simulink model "prattico_simscape_phase_b"  (R2025b)
settings: Solver=ode23t  StartTime=0.0  StopTime=1  MaxStep=3e-6  RelTol=1e-4  AbsTol=1e-5
libraries: fl_lib x24, nesl_utility x14, simulink x8, batteryecm_lib x1, slpidlib x1, ee_lib x1
settings Model: Creator=oakir  LastModifiedBy=oakir
settings DataIOCC: SignalLogging=off  ReturnWorkspaceOutputs=off

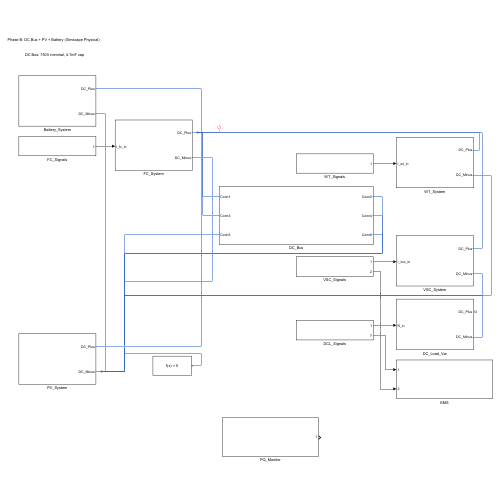
[thumbnail: Simulink's stored preview of the top-level diagram]
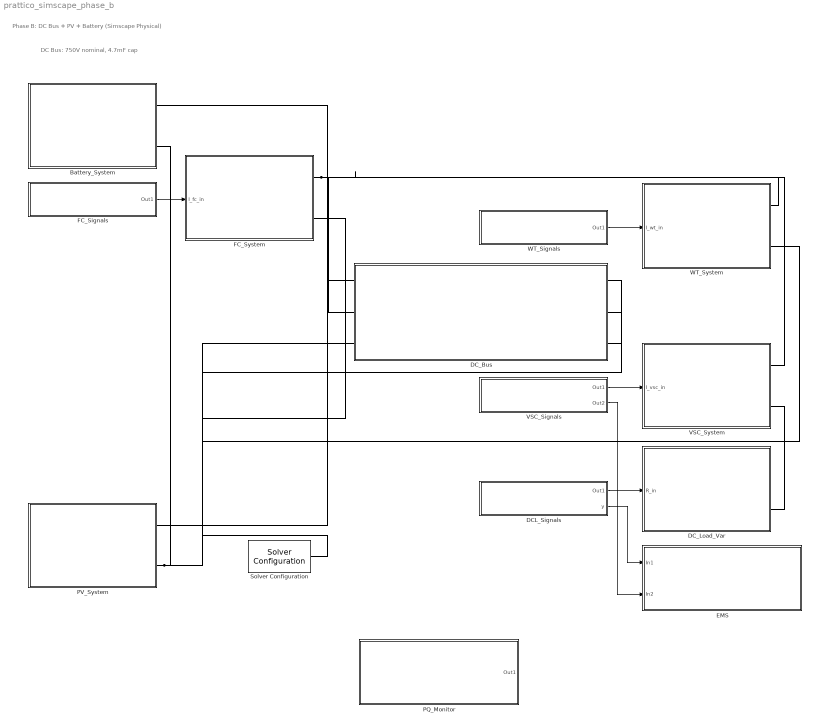
== system prattico_simscape_phase_b ==
  note: DC Bus: 750V nominal, 4.7mF cap
  note: Phase B: DC Bus + PV + Battery (Simscape Physical)
  Battery_System : Subsystem
  DCL_Signals : Subsystem
  DC_Bus : Subsystem
  DC_Load_Var : Subsystem
  EMS : Subsystem
  FC_Signals : Subsystem
  FC_System : Subsystem
  PQ_Monitor : Subsystem
  PV_System : Subsystem
  Solver Configuration : nesl_utility/Solver Configuration  PhysicalDomain=network_engine_domain  SubClassName=solver  LeftPortType=input  RightPortType=generic  Tones=[]  Harmonics=[]  SimulateNoise=off  Profile=off  UseLocalSampling=off  EnableSwitchedLinearOptims=on  FrequencyDomain=off  UseCCode=off  RelTol=0.001  AbsTol=0.001  MinStep=1e-09  ToWorkspace=off  RevertToSquareIcSolve=off  NumHomotopyIterations=100  PhasorMode=off  PhasorModeNumHarmonics=1  ConsistencySolver=NEWTON_XTOL_AFTER_FTOL  IndexReductionMethod=DerivativeReplacement  DoDC=off  ResidualTolerance=1e-09  ConsistencyTolSource=GLOBAL  ConsistencyAbsTol=0.001  ConsistencyRelTol=0.001  ConsistencyTolFactor=0.001  UseLocalSolver=off  LocalSolverChoice=NE_BACKWARD_EULER_ADVANCER  ResolveIndetEquations=on  FunctionEvalNumThread=1  LocalSolverSampleTime=0.001  DoFixedCost=off  MaxNonlinIter=3  MaxModeIter=2  ComputeImpulses=off  ImpulseIterations=2  LinearAlgebra=auto  LinearAlgebraNumThread=0  EquationFormulation=NE_TIME_EF  DelaysMemoryBudget=1024  AutomaticFiltering=on  FilteringTimeConstant=0.001  PartitionStorageMethod=AS_NEEDED  PartitionMemoryBudget=1024  PartitionMethod=ROBUST  MultibodyUseLocalSolver=off  MultibodyLocalSolverChoice=ODE1  MultibodyLocalSolverSampleTime=0.001
  VSC_Signals : Subsystem
  VSC_System : Subsystem
  WT_Signals : Subsystem
  WT_System : Subsystem
  wires:
  FC_Signals/1(Out1) -> FC_System/1(I_fc_in)
  DCL_Signals/2(y) -> EMS/1(In1)
  DCL_Signals/1(Out1) -> DC_Load_Var/1(R_in)
  WT_Signals/1(Out1) -> WT_System/1(I_wt_in)
  VSC_Signals/2(Out2) -> EMS/2(In2)
  VSC_Signals/1(Out1) -> VSC_System/1(I_vsc_in)
  connections:
  FC_System/RConn1 -- VSC_System/RConn1 -- Battery_System/RConn1 -- WT_System/RConn1 -- DC_Bus/LConn2 -- DC_Bus/LConn1 -- PV_System/RConn1
  DC_Bus/RConn2 -- Solver Configuration/RConn1 -- PV_System/RConn2 -- FC_System/RConn2 -- WT_System/RConn2 -- VSC_System/RConn2 -- DC_Load_Var/RConn2 -- Battery_System/RConn2 -- DC_Bus/RConn3 -- DC_Bus/LConn3 -- DC_Bus/RConn1

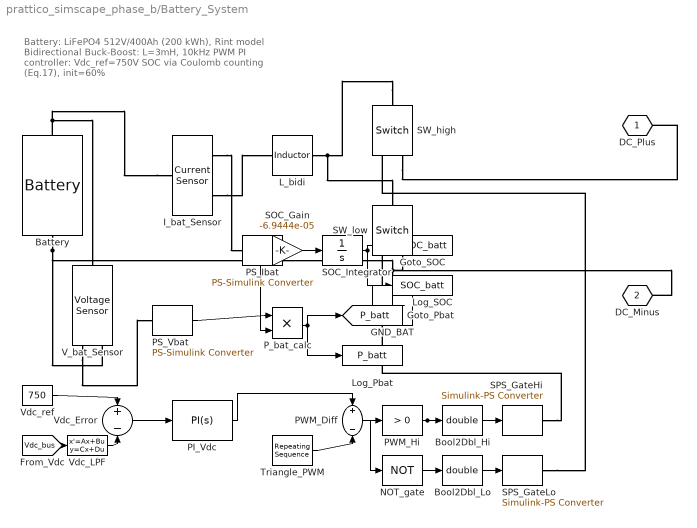
== system prattico_simscape_phase_b/Battery_System ==
  note: Battery: LiFePO4 512V/400Ah (200 kWh), Rint model
      | Bidirectional Buck-Boost: L=3mH, 10kHz PWM
      | PI controller: Vdc_ref=750V
      | SOC via Coulomb counting (Eq.17), init=60%
  Battery : batteryecm_lib/Battery  Vnom=512 V  prm_dir=simscape.enum.battery.prm_dir.disabled  R1_dis=2 Ohm  R1_ch=2 Ohm  R1=0.04 Ohm  prm_AH=simscape.enum.battery.prm_AH.infinite  AH=400 A*hr  V1=480 V  AH1=360 A*hr  prm_R2=simscape.enum.battery.prm_R2.disabled  R2=2000 Ohm  Tmeas=298.15 K  charge_measurement_port=simscape.enum.battery.enable.no  prm_dyn=simscape.enum.battery.prm_dyn.off  Rp1=0.005 Ohm  tau1=30 s  Rp2=0.005 Ohm  tau2=30 s  Rp3=0.005 Ohm  tau3=30 s  Rp4=0.005 Ohm  tau4=30 s  Rp5=0.005 Ohm  tau5=30 s  prm_fade=simscape.enum.battery.prm_fade.disabled  N_fade=100  AH_fade=45 A*hr  R1_fade=2.02 Ohm  R1_ch_fade=2.02 Ohm  V1_fade=10.35 V  prm_age=simscape.enum.battery.prm_age.disabled  prm_age_OCV=simscape.enum.battery.prm_age_OCV.OCV  OCV_age=0.9  SOC_age=60  Tmeas_age=298.15 K  delta_time_age_vec=[0] d  temperature_age_vec=[273] K  OCV_scaling_age=2.2134e6  OCV_offset_age=1.632e6  temp_exp_age=0.515833569 V  t_exp_age=0.75  Vnom_T2=12 V  R1_T2=2.2 Ohm  R1_T2_dis=2.2 Ohm  R1_T2_ch=2.2 Ohm  V1_T2=11.4 V  R2_T2=2200 Ohm  Rp1_T2=0.005 Ohm  tau1_T2=30 s  Rp2_T2=0.005 Ohm  tau2_T2=30 s  Rp3_T2=0.005 Ohm  tau3_T2=30 s  Rp4_T2=0.005 Ohm  tau4_T2=30 s  Rp5_T2=0.005 Ohm  tau5_T2=30 s  Tmeas2=273.15 K  thermal_port=simscape.enum.thermaleffects.omit  thermal_mass=30000 J/K  i_specify=off  i_priority=None  i=0 A  i_nominal_specify=off  i_nominal_value=1  i_nominal_unit=A  v_specify=off  v_priority=None  v=0 V  v_nominal_specify=off  v_nominal_value=1  v_nominal_unit=V  charge_specify=off  charge_priority=High  charge=50 A*hr  charge_nominal_specify=off  charge_nominal_value=1  charge_nominal_unit=A*hr  num_cycles_specify=off  num_cycles_priority=High  num_cycles=0  num_cycles_nominal_specify=off  num_cycles_nominal_value=1  num_cycles_nominal_unit=1  temperature_specify=off  temperature_priority=High  temperature=298.15 K  temperature_nominal_specify=off  temperature_nominal_value=1  temperature_nominal_unit=K
  Bool2Dbl_Hi : DataTypeConversion  OutDataTypeStr=double  SaturateOnIntegerOverflow=off  RndMeth=Floor
  Bool2Dbl_Lo : DataTypeConversion  OutDataTypeStr=double  SaturateOnIntegerOverflow=off  RndMeth=Floor
  GND_BAT : fl_lib/Electrical/Electrical Elements/Electrical Reference
  I_bat_Sensor : fl_lib/Electrical/Electrical Sensors/Current Sensor
  L_bidi : fl_lib/Electrical/Electrical Elements/Inductor  l=3e-3 H  r=0 Ohm  g=1e-9 1/Ohm  i_specify=off  i_priority=None  i=0 A  i_nominal_specify=off  i_nominal_value=1  i_nominal_unit=A  v_specify=off  v_priority=None  v=0 V  v_nominal_specify=off  v_nominal_value=1  v_nominal_unit=V  i_L_specify=off  i_L_priority=High  i_L=0 A  i_L_nominal_specify=off  i_L_nominal_value=1  i_L_nominal_unit=A
  Log_Pbat : ToWorkspace  VariableName=P_batt  SaveFormat=Timeseries  SampleTime=-1
  Log_SOC : ToWorkspace  VariableName=SOC_batt  SaveFormat=Timeseries  SampleTime=-1
  NOT_gate : Logic  Operator=NOT  AllPortsSameDT=off  OutDataTypeStr=boolean
  PI_Vdc : slpidlib/PID Controller  Controller=PI  Form=Parallel  TimeDomain=Continuous-time  UseExternalTs=off  SampleTime=-1  IntegratorMethod=Forward Euler  FilterMethod=Forward Euler  ControllerParametersSource=internal  P=0.0001  I=0.02  UseKiTs=off  D=0  UseExternalDerivativeSource=off  N=100  UseFilter=on  TunerSelectOption=Transfer Function Based (PID Tuner App)  InitialConditionSource=internal  InitialConditionForIntegrator=0.32  InitialConditionForFilter=0  DifferentiatorICPrevScaledInput=0  ExternalReset=none  TrackingMode=off  Kt=1  LimitOutput=off  SatLimitsSource=internal  UpperSaturationLimit=0.45  LowerSaturationLimit=0.05  LinearizeAsGain=on  AntiWindupMode=none  Kb=1  LimitIntegrator=off  UpperIntegratorSaturationLimit=inf  LowerIntegratorSaturationLimit=-inf  POutMin=[]  POutMax=[]  IOutMin=[]  IOutMax=[]  DOutMin=[]  DOutMax=[]  NOutMin=[]  NOutMax=[]  SumOutMin=[]  SumOutMax=[]  SaturationOutMin=[]  SaturationOutMax=[]  PParamMin=[]  PParamMax=[]  IParamMin=[]  IParamMax=[]  DParamMin=[]  DParamMax=[]  NParamMin=[]  NParamMax=[]  KbParamMin=[]  KbParamMax=[]  KtParamMin=[]  KtParamMax=[]  KbOutMin=[]  KbOutMax=[]  KtOutMin=[]  KtOutMax=[]  IntegratorOutMin=[]  IntegratorOutMax=[]  FilterOutMin=[]  FilterOutMax=[]  SumI1OutMin=[]  SumI1OutMax=[]  SumI2OutMin=[]  SumI2OutMax=[]  SumI3OutMin=[]  SumI3OutMax=[]  SumI4OutMin=[]  SumI4OutMax=[]  SumDOutMin=[]  SumDOutMax=[]  DifferentiatorOutMin=[]  DifferentiatorOutMax=[]  FilterDiffOutCoefMin=[]  FilterDiffOutCoefMax=[]  ReciprocalOutMin=[]  ReciprocalOutMax=[]  SumDenOutMin=[]  SumDenOutMax=[]  SumNumOutMin=[]  SumNumOutMax=[]  DivideOutMin=[]  DivideOutMax=[]  UdiffTsProdOutMin=[]  UdiffTsProdOutMax=[]  NTsProdOutMin=[]  NTsProdOutMax=[]  UintegralTsProdOutMin=[]  UintegralTsProdOutMax=[]  UngainTsProdOutMin=[]  UngainTsProdOutMax=[]  ClampingZeroOutDataTypeStr=Inherit: Inherit via back propagation  ClampingZeroOutMin=[]  ClampingZeroOutMax=[]  FilterDenConstantOutDataTypeStr=Inherit: Inherit via back propagation  FilterDenConstantOutMin=[]  FilterDenConstantOutMax=[]  PCopyOutDataTypeStr=Inherit: Inherit via back propagation  PCopyOutMin=[]  PCopyOutMax=[]  NCopyOutDataTypeStr=Inherit: Inherit via back propagation  NCopyOutMin=[]  NCopyOutMax=[]  IntegratorContinuousStateAttributes=''  IntegratorStateMustResolveToSignalObject=off  IntegratorRTWStateStorageClass=Auto  FilterContinuousStateAttributes=''  FilterStateMustResolveToSignalObject=off  FilterRTWStateStorageClass=Auto  ParallelPVariant=InternalParameters  IdealPVariant=Disabled  IVariant=InternalParameters  DVariant=Disabled  IntegratorVariant=Continuous  SatVariant=Disabled  AWVariant=Passthrough  PCopyVariant=Disabled  TRVariant=Disabled  FdbkBlocksVariant=Forward  IdealPFdbkVariant=Disabled  SatFdbkVariant=Disabled  DerivativeFilterVariant=Disabled  NVariant=Disabled  NCopyVariant=Disabled_SignalSpec  FilterICVariant=Disabled  IntegratorICVariant=InternalICs  ExternalResetVariant=Disabled  TRSumVariant=Passthrough  SumFdbkVariant=Disabled  SumVariant=Sum_PI  TsampFilterVariant=InternalTs  TsampNgainVariant=Passthrough  TsampIntegralVariant=Disabled_SignalSpec  ExternalSaturationOutDataTypeStr=Inherit: Same as second input  DerivativeSourceVariant=Disabled  PreIntVariant=InternalPreInt
  PS_Ibat : nesl_utility/PS-Simulink Converter  PhysicalDomain=network_engine_domain  SubClassName=ps_output  LeftPortType=input  RightPortType=output  PseudoPeriodic=off  Frequencies=[]  VectorFormat=inherit  Unit=inherit  AffineConversion=off
  PS_Vbat : nesl_utility/PS-Simulink Converter  PhysicalDomain=network_engine_domain  SubClassName=ps_output  LeftPortType=input  RightPortType=output  PseudoPeriodic=off  Frequencies=[]  VectorFormat=inherit  Unit=inherit  AffineConversion=off
  PWM_Diff : Sum  Inputs=+-
  PWM_Hi : simulink/Logic and Bit Operations/Compare To Zero  relop=>  OutDataTypeStr=boolean
  P_bat_calc : Product
  SOC_Gain : Gain  Gain=-6.9444e-05
  SOC_Integrator : Integrator  InitialCondition=60  UpperSaturationLimit=100  LowerSaturationLimit=0
  SPS_GateHi : nesl_utility/Simulink-PS Converter  PhysicalDomain=network_engine_domain  SubClassName=ps_input  LeftPortType=input  RightPortType=output  PseudoPeriodic=off  Frequencies=[]  NoiseDistribution=none  NoiseParameters=[]  Unit=1  AffineConversion=off  FilteringAndDerivatives=provide  SimscapeFilterOrder=1  InputFilterTimeConstant=1e-7  UdotUserProvided=0
  SPS_GateLo : nesl_utility/Simulink-PS Converter  PhysicalDomain=network_engine_domain  SubClassName=ps_input  LeftPortType=input  RightPortType=output  PseudoPeriodic=off  Frequencies=[]  NoiseDistribution=none  NoiseParameters=[]  Unit=1  AffineConversion=off  FilteringAndDerivatives=provide  SimscapeFilterOrder=1  InputFilterTimeConstant=1e-7  UdotUserProvided=0
  SW_high : fl_lib/Electrical/Electrical Elements/Switch  R_closed=0.01 Ohm  G_open=1e-8 1/Ohm  Threshold=0.5  i_specify=off  i_priority=None  i=0 A  i_nominal_specify=off  i_nominal_value=1  i_nominal_unit=A  v_specify=off  v_priority=None  v=0 V  v_nominal_specify=off  v_nominal_value=1  v_nominal_unit=V
  SW_low : fl_lib/Electrical/Electrical Elements/Switch  R_closed=0.01 Ohm  G_open=1e-8 1/Ohm  Threshold=0.5  i_specify=off  i_priority=None  i=0 A  i_nominal_specify=off  i_nominal_value=1  i_nominal_unit=A  v_specify=off  v_priority=None  v=0 V  v_nominal_specify=off  v_nominal_value=1  v_nominal_unit=V
  Triangle_PWM : simulink/Sources/Repeating Sequence  rep_seq_t=[0 5e-5 1e-4]  rep_seq_y=[0 1 0]
  V_bat_Sensor : fl_lib/Electrical/Electrical Sensors/Voltage Sensor
  Vdc_Error : Sum  Inputs=+-
  Vdc_LPF : StateSpace  A=-200  B=200  D=0  InitialCondition=750
  Vdc_ref : Constant  Value=750
  DC_Plus : PMIOPort  Side=Right
  DC_Minus : PMIOPort  Port=2  Side=Right
  tag scope: P_batt=global, SOC_batt=global
  wires:
  PS_Ibat/1 -> SOC_Gain/1, P_bat_calc/2
  SOC_Gain/1 -> SOC_Integrator/1
  SOC_Integrator/1 -> [SOC_batt], Log_SOC/1
  PS_Vbat/1 -> P_bat_calc/1
  P_bat_calc/1 -> [P_batt], Log_Pbat/1
  Vdc_ref/1 -> Vdc_Error/1
  [Vdc_bus] -> Vdc_LPF/1
  Vdc_LPF/1 -> Vdc_Error/2
  Vdc_Error/1 -> PI_Vdc/1
  PI_Vdc/1 -> PWM_Diff/1
  Triangle_PWM/1 -> PWM_Diff/2
  PWM_Diff/1 -> PWM_Hi/1
  PWM_Hi/1 -> Bool2Dbl_Hi/1, NOT_gate/1
  Bool2Dbl_Hi/1 -> SPS_GateHi/1
  NOT_gate/1 -> Bool2Dbl_Lo/1
  Bool2Dbl_Lo/1 -> SPS_GateLo/1
  connections:
  I_bat_Sensor/LConn1 -- Battery/LConn1 -- V_bat_Sensor/LConn1
  I_bat_Sensor/RConn2 -- L_bidi/LConn1
  Battery/RConn1 -- V_bat_Sensor/RConn2 -- SW_low/RConn2 -- GND_BAT/LConn1 -- DC_Minus/RConn1
  SW_high/LConn1 -- L_bidi/RConn1 -- SW_low/LConn1
  SW_high/RConn2 -- DC_Plus/RConn1
  SPS_GateHi/RConn1 -- SW_low/RConn1
  SPS_GateLo/RConn1 -- SW_high/RConn1
  I_bat_Sensor/RConn1 -- PS_Ibat/LConn1
  V_bat_Sensor/RConn1 -- PS_Vbat/LConn1

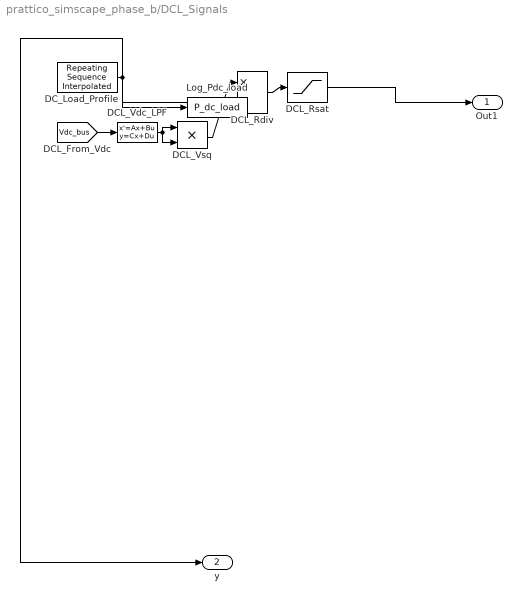
== system prattico_simscape_phase_b/DCL_Signals ==
  DCL_Rdiv : Product  Inputs=*/
  DCL_Rsat : Saturate  UpperLimit=1e6  LowerLimit=1
  DCL_Vdc_LPF : StateSpace  A=-200  B=200  D=0  InitialCondition=750
  DCL_Vsq : Product  Inputs=**
  DC_Load_Profile : simulink/Sources/Repeating Sequence Interpolated  OutValues=[1500 1500 6000 12000 12000 12000 15000 12000 10000 6000 3000 1500 1500]  TimeValues=[0 7 7.5 8.5 9 11 14 15 17 19 20 22 24]  LookUpMeth=Interpolation-Use End Values  tsamp=0.01  OutMin=[]  OutMax=[]  OutDataTypeStr=double  OutputDataTypeScalingMode=double  OutDataType=fixdt(0,8)  OutScaling=2^-10
  Log_Pdc_load : ToWorkspace  VariableName=P_dc_load  SaveFormat=Timeseries  SampleTime=-1
  Out1 : Outport
  y : Outport  Port=2
  wires:
  DC_Load_Profile/1 -> y/1, Log_Pdc_load/1, DCL_Rdiv/2
  DCL_Vsq/1 -> DCL_Rdiv/1
  DCL_Vdc_LPF/1 -> DCL_Vsq/1, DCL_Vsq/2
  [Vdc_bus] -> DCL_Vdc_LPF/1
  DCL_Rdiv/1 -> DCL_Rsat/1
  DCL_Rsat/1 -> Out1/1

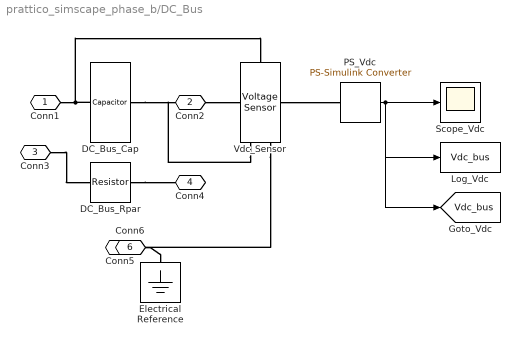
== system prattico_simscape_phase_b/DC_Bus ==
  DC_Bus_Cap : fl_lib/Electrical/Electrical Elements/Capacitor  c=4.7e-3 F  r=1e-6 Ohm  g=0 1/Ohm  i_specify=off  i_priority=None  i=0 A  i_nominal_specify=off  i_nominal_value=1  i_nominal_unit=A  v_specify=off  v_priority=None  v=750 V  v_nominal_specify=off  v_nominal_value=1  v_nominal_unit=V  vc_specify=off  vc_priority=High  vc=0 V  vc_nominal_specify=off  vc_nominal_value=1  vc_nominal_unit=V
  DC_Bus_Rpar : fl_lib/Electrical/Electrical Elements/Resistor  R=1e4 Ohm  i_specify=off  i_priority=None  i=0 A  i_nominal_specify=off  i_nominal_value=1  i_nominal_unit=A  v_specify=off  v_priority=None  v=0 V  v_nominal_specify=off  v_nominal_value=1  v_nominal_unit=V
  Electrical Reference : fl_lib/Electrical/Electrical Elements/Electrical Reference
  Log_Vdc : ToWorkspace  VariableName=Vdc_bus  SaveFormat=Timeseries  SampleTime=-1
  PS_Vdc : nesl_utility/PS-Simulink Converter  PhysicalDomain=network_engine_domain  SubClassName=ps_output  LeftPortType=input  RightPortType=output  PseudoPeriodic=off  Frequencies=[]  VectorFormat=inherit  Unit=inherit  AffineConversion=off
  Scope_Vdc : Scope
  Vdc_Sensor : fl_lib/Electrical/Electrical Sensors/Voltage Sensor
  Conn1 : PMIOPort  Side=Left
  Conn2 : PMIOPort  Port=2  Side=Right
  Conn3 : PMIOPort  Port=3  Side=Left
  Conn4 : PMIOPort  Port=4  Side=Right
  Conn5 : PMIOPort  Port=5  Side=Left
  Conn6 : PMIOPort  Port=6  Side=Right
  tag scope: Vdc_bus=global
  wires:
  PS_Vdc/1 -> Scope_Vdc/1, Log_Vdc/1, [Vdc_bus]
  connections:
  Conn3/RConn1 -- DC_Bus_Rpar/LConn1
  DC_Bus_Rpar/RConn1 -- Conn4/RConn1
  Vdc_Sensor/RConn1 -- PS_Vdc/LConn1
  Vdc_Sensor/RConn2 -- Conn6/RConn1
  DC_Bus_Cap/RConn1 -- Conn2/RConn1
  Conn1/RConn1 -- Vdc_Sensor/LConn1 -- DC_Bus_Cap/LConn1
  Conn5/RConn1 -- Electrical Reference/LConn1

== system prattico_simscape_phase_b/DC_Load_Var ==
  R_in : Inport
  SPS_R : nesl_utility/Simulink-PS Converter  PhysicalDomain=network_engine_domain  SubClassName=ps_input  LeftPortType=input  RightPortType=output  PseudoPeriodic=off  Frequencies=[]  NoiseDistribution=none  NoiseParameters=[]  Unit=1  AffineConversion=off  FilteringAndDerivatives=provide  SimscapeFilterOrder=1  InputFilterTimeConstant=0.001  UdotUserProvided=0
  VR_DC : fl_lib/Electrical/Electrical Elements/Variable Resistor  Rmin=0 Ohm  thermalEnable=false  thermal_mass=1 J/K  i_specify=off  i_priority=None  i=0 A  i_nominal_specify=off  i_nominal_value=1  i_nominal_unit=A  v_specify=off  v_priority=None  v=0 V  v_nominal_specify=off  v_nominal_value=1  v_nominal_unit=V  T_specify=off  T_priority=None  T=300 K  T_nominal_specify=off  T_nominal_value=1  T_nominal_unit=K
  DC_Plus : PMIOPort  Side=Right
  DC_Minus : PMIOPort  Port=2  Side=Right
  wires:
  R_in/1 -> SPS_R/1
  connections:
  VR_DC/LConn1 -- DC_Plus/RConn1
  VR_DC/RConn1 -- DC_Minus/RConn1

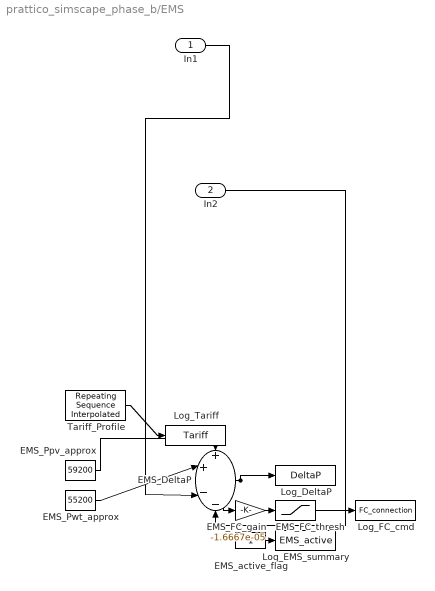
== system prattico_simscape_phase_b/EMS ==
  In1 : Inport
  In2 : Inport  Port=2
  EMS_DeltaP : Sum  Inputs=++--
  EMS_FC_gain : Gain  Gain=-1.6667e-05
  EMS_FC_thresh : Saturate  UpperLimit=1  LowerLimit=0
  EMS_Ppv_approx : Constant  Value=59200
  EMS_Pwt_approx : Constant  Value=55200
  EMS_active_flag : Constant
  Log_DeltaP : ToWorkspace  VariableName=DeltaP  SaveFormat=Timeseries  SampleTime=-1
  Log_EMS_summary : ToWorkspace  VariableName=EMS_active  SaveFormat=Timeseries  SampleTime=-1
  Log_FC_cmd : ToWorkspace  VariableName=FC_connection  SaveFormat=Timeseries  SampleTime=-1
  Log_Tariff : ToWorkspace  VariableName=Tariff  SaveFormat=Timeseries  SampleTime=-1
  Tariff_Profile : simulink/Sources/Repeating Sequence Interpolated  OutValues=[0.05 0.05 0.08 0.1 0.12 0.1 0.15 0.15 0.1 0.05]  TimeValues=[0 6 7 9 11 17 19 21 22 24]  LookUpMeth=Interpolation-Use End Values  tsamp=0.01  OutMin=[]  OutMax=[]  OutDataTypeStr=double  OutputDataTypeScalingMode=double  OutDataType=fixdt(0,8)  OutScaling=2^-10
  wires:
  EMS_Ppv_approx/1 -> EMS_DeltaP/1
  EMS_DeltaP/1 -> Log_DeltaP/1, EMS_FC_gain/1
  Tariff_Profile/1 -> Log_Tariff/1
  In2/1 -> EMS_DeltaP/4
  EMS_FC_gain/1 -> EMS_FC_thresh/1
  EMS_FC_thresh/1 -> Log_FC_cmd/1
  EMS_Pwt_approx/1 -> EMS_DeltaP/2
  EMS_active_flag/1 -> Log_EMS_summary/1
  In1/1 -> EMS_DeltaP/3

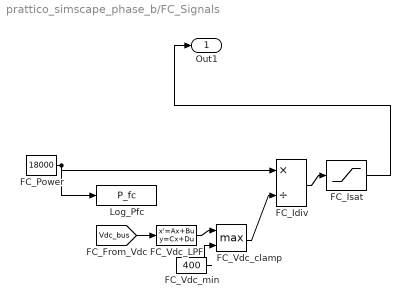
== system prattico_simscape_phase_b/FC_Signals ==
  FC_Idiv : Product  Inputs=*/
  FC_Isat : Saturate  UpperLimit=50  LowerLimit=0
  FC_Power : Constant  Value=18000
  FC_Vdc_LPF : StateSpace  A=-200  B=200  D=0  InitialCondition=750
  FC_Vdc_clamp : MinMax  Function=max  Inputs=2
  FC_Vdc_min : Constant  Value=400
  Log_Pfc : ToWorkspace  VariableName=P_fc  SaveFormat=Timeseries  SampleTime=-1
  Out1 : Outport
  wires:
  FC_Isat/1 -> Out1/1
  FC_Vdc_clamp/1 -> FC_Idiv/2
  FC_Power/1 -> FC_Idiv/1, Log_Pfc/1
  FC_Vdc_min/1 -> FC_Vdc_clamp/2
  [Vdc_bus] -> FC_Vdc_LPF/1
  FC_Vdc_LPF/1 -> FC_Vdc_clamp/1
  FC_Idiv/1 -> FC_Isat/1

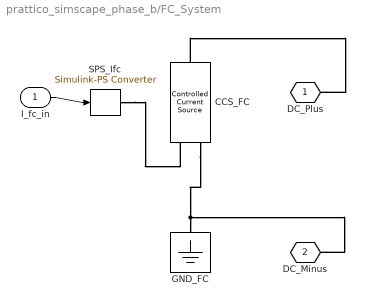
== system prattico_simscape_phase_b/FC_System ==
  I_fc_in : Inport
  CCS_FC : fl_lib/Electrical/Electrical Sources/Controlled Current Source
  GND_FC : fl_lib/Electrical/Electrical Elements/Electrical Reference
  SPS_Ifc : nesl_utility/Simulink-PS Converter  PhysicalDomain=network_engine_domain  SubClassName=ps_input  LeftPortType=input  RightPortType=output  PseudoPeriodic=off  Frequencies=[]  NoiseDistribution=none  NoiseParameters=[]  Unit=1  AffineConversion=off  FilteringAndDerivatives=provide  SimscapeFilterOrder=1  InputFilterTimeConstant=0.001  UdotUserProvided=0
  DC_Plus : PMIOPort  Side=Right
  DC_Minus : PMIOPort  Port=2  Side=Right
  wires:
  I_fc_in/1 -> SPS_Ifc/1
  connections:
  SPS_Ifc/RConn1 -- CCS_FC/RConn1
  CCS_FC/LConn1 -- DC_Plus/RConn1
  GND_FC/LConn1 -- CCS_FC/RConn2 -- DC_Minus/RConn1

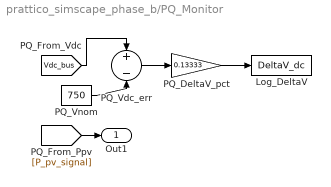
== system prattico_simscape_phase_b/PQ_Monitor ==
  Log_DeltaV : ToWorkspace  VariableName=DeltaV_dc  SaveFormat=Timeseries  SampleTime=-1
  PQ_DeltaV_pct : Gain  Gain=0.13333
  PQ_Vdc_err : Sum  Inputs=+-
  PQ_Vnom : Constant  Value=750
  Out1 : Outport
  wires:
  PQ_Vdc_err/1 -> PQ_DeltaV_pct/1
  [P_pv_signal] -> Out1/1
  PQ_DeltaV_pct/1 -> Log_DeltaV/1
  [Vdc_bus] -> PQ_Vdc_err/1
  PQ_Vnom/1 -> PQ_Vdc_err/2

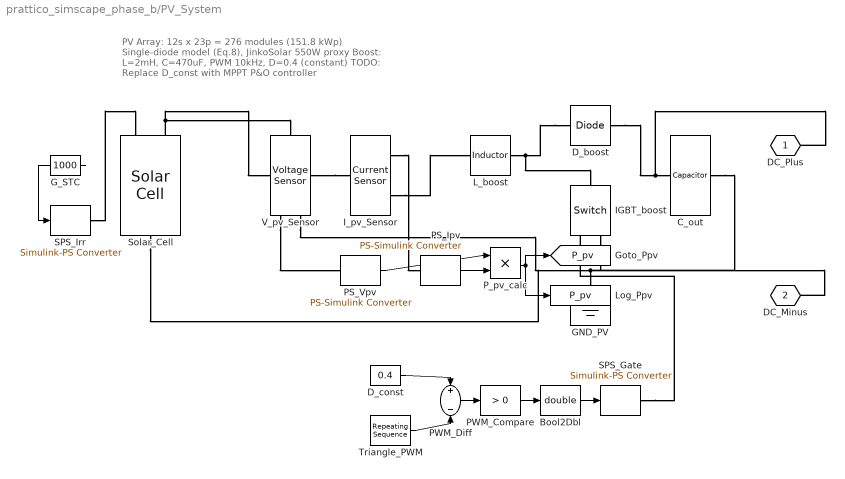
== system prattico_simscape_phase_b/PV_System ==
  note: PV Array: 12s x 23p = 276 modules (151.8 kWp)
      | Single-diode model (Eq.8), JinkoSolar 550W proxy
      | Boost: L=2mH, C=470uF, PWM 10kHz, D=0.4 (constant)
      | TODO: Replace D_const with MPPT P&O controller
  Bool2Dbl : DataTypeConversion  OutDataTypeStr=double  SaturateOnIntegerOverflow=off  RndMeth=Floor
  C_out : fl_lib/Electrical/Electrical Elements/Capacitor  c=470e-6 F  r=1e-6 Ohm  g=0 1/Ohm  i_specify=off  i_priority=None  i=0 A  i_nominal_specify=off  i_nominal_value=1  i_nominal_unit=A  v_specify=off  v_priority=None  v=750 V  v_nominal_specify=off  v_nominal_value=1  v_nominal_unit=V  vc_specify=off  vc_priority=High  vc=0 V  vc_nominal_specify=off  vc_nominal_value=1  vc_nominal_unit=V
  D_boost : fl_lib/Electrical/Electrical Elements/Diode  Vf=0.6 V  Ron=0.3 Ohm  Goff=1e-8 1/Ohm  i_specify=off  i_priority=None  i=0 A  i_nominal_specify=off  i_nominal_value=1  i_nominal_unit=A  v_specify=off  v_priority=None  v=0 V  v_nominal_specify=off  v_nominal_value=1  v_nominal_unit=V
  D_const : Constant  Value=0.4
  GND_PV : fl_lib/Electrical/Electrical Elements/Electrical Reference
  G_STC : Constant  Value=1000
  IGBT_boost : fl_lib/Electrical/Electrical Elements/Switch  R_closed=0.01 Ohm  G_open=1e-8 1/Ohm  Threshold=0.5  i_specify=off  i_priority=None  i=0 A  i_nominal_specify=off  i_nominal_value=1  i_nominal_unit=A  v_specify=off  v_priority=None  v=0 V  v_nominal_specify=off  v_nominal_value=1  v_nominal_unit=V
  I_pv_Sensor : fl_lib/Electrical/Electrical Sensors/Current Sensor
  L_boost : fl_lib/Electrical/Electrical Elements/Inductor  l=2e-3 H  r=0 Ohm  g=1e-9 1/Ohm  i_specify=off  i_priority=None  i=0 A  i_nominal_specify=off  i_nominal_value=1  i_nominal_unit=A  v_specify=off  v_priority=None  v=0 V  v_nominal_specify=off  v_nominal_value=1  v_nominal_unit=V  i_L_specify=off  i_L_priority=High  i_L=0 A  i_L_nominal_specify=off  i_L_nominal_value=1  i_L_nominal_unit=A
  Log_Ppv : ToWorkspace  VariableName=P_pv  SaveFormat=Timeseries  SampleTime=-1
  PS_Ipv : nesl_utility/PS-Simulink Converter  PhysicalDomain=network_engine_domain  SubClassName=ps_output  LeftPortType=input  RightPortType=output  PseudoPeriodic=off  Frequencies=[]  VectorFormat=inherit  Unit=inherit  AffineConversion=off
  PS_Vpv : nesl_utility/PS-Simulink Converter  PhysicalDomain=network_engine_domain  SubClassName=ps_output  LeftPortType=input  RightPortType=output  PseudoPeriodic=off  Frequencies=[]  VectorFormat=inherit  Unit=inherit  AffineConversion=off
  PWM_Compare : simulink/Logic and Bit Operations/Compare To Zero  relop=>  OutDataTypeStr=boolean
  PWM_Diff : Sum  Inputs=+-
  P_pv_calc : Product
  SPS_Gate : nesl_utility/Simulink-PS Converter  PhysicalDomain=network_engine_domain  SubClassName=ps_input  LeftPortType=input  RightPortType=output  PseudoPeriodic=off  Frequencies=[]  NoiseDistribution=none  NoiseParameters=[]  Unit=1  AffineConversion=off  FilteringAndDerivatives=provide  SimscapeFilterOrder=1  InputFilterTimeConstant=0.001  UdotUserProvided=0
  SPS_Irr : nesl_utility/Simulink-PS Converter  PhysicalDomain=network_engine_domain  SubClassName=ps_input  LeftPortType=input  RightPortType=output  PseudoPeriodic=off  Frequencies=[]  NoiseDistribution=none  NoiseParameters=[]  Unit=1  AffineConversion=off  FilteringAndDerivatives=provide  SimscapeFilterOrder=1  InputFilterTimeConstant=0.001  UdotUserProvided=0
  Solar_Cell : ee_lib/Sources/Solar Cell  prm=ee.enum.sources.solar_cell_prm.datasheet  Isc=7.34 A  Voc=0.6 V  Is=1e-6 A  Is2=0 A  Iph=7.34 A  Ir0=1000 W/m^2  ec=1.5  N2=2  Rs=0 Ohm  Rp=inf Ohm  N_series=864  N_parallel=23  TIPH1=0 1/K  EG=1.11 eV  TXIS1=3  TXIS2=3  TRS1=0  TRP1=0  Tmeas=25 degC  TFIXED=25 degC  thermal_mass=100 J/K  initial_temperature=25 degC
  Triangle_PWM : simulink/Sources/Repeating Sequence  rep_seq_t=[0 5e-5 1e-4]  rep_seq_y=[0 1 0]
  V_pv_Sensor : fl_lib/Electrical/Electrical Sensors/Voltage Sensor
  DC_Plus : PMIOPort  Side=Right
  DC_Minus : PMIOPort  Port=2  Side=Right
  tag scope: P_pv=global
  wires:
  G_STC/1 -> SPS_Irr/1
  PS_Vpv/1 -> P_pv_calc/1
  PS_Ipv/1 -> P_pv_calc/2
  P_pv_calc/1 -> [P_pv], Log_Ppv/1
  D_const/1 -> PWM_Diff/1
  Triangle_PWM/1 -> PWM_Diff/2
  PWM_Diff/1 -> PWM_Compare/1
  PWM_Compare/1 -> Bool2Dbl/1
  Bool2Dbl/1 -> SPS_Gate/1
  connections:
  SPS_Irr/RConn1 -- Solar_Cell/LConn1
  I_pv_Sensor/LConn1 -- Solar_Cell/LConn2 -- V_pv_Sensor/LConn1
  Solar_Cell/RConn1 -- V_pv_Sensor/RConn2 -- IGBT_boost/RConn2 -- C_out/RConn1 -- GND_PV/LConn1 -- DC_Minus/RConn1
  V_pv_Sensor/RConn1 -- PS_Vpv/LConn1
  I_pv_Sensor/RConn2 -- L_boost/LConn1
  I_pv_Sensor/RConn1 -- PS_Ipv/LConn1
  D_boost/LConn1 -- L_boost/RConn1 -- IGBT_boost/LConn1
  C_out/LConn1 -- D_boost/RConn1 -- DC_Plus/RConn1
  SPS_Gate/RConn1 -- IGBT_boost/RConn1

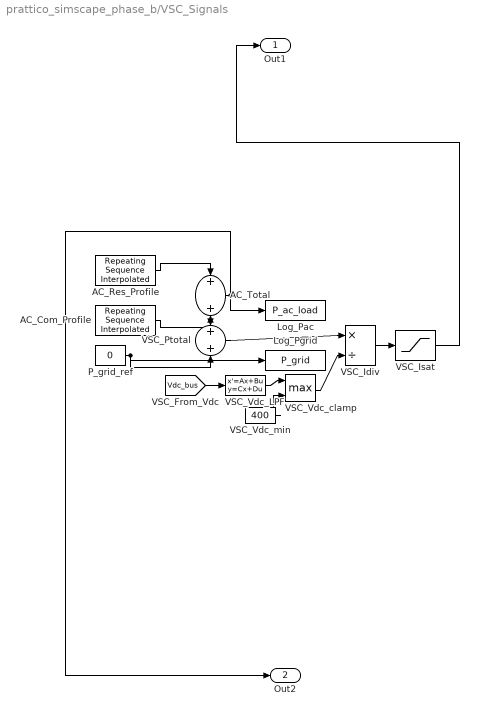
== system prattico_simscape_phase_b/VSC_Signals ==
  AC_Com_Profile : simulink/Sources/Repeating Sequence Interpolated  OutValues=[5000 5000 35000 35000 45000 35000 15000 5000]  TimeValues=[0 7 8 12 13 18 20 24]  LookUpMeth=Interpolation-Use End Values  tsamp=0.01  OutMin=[]  OutMax=[]  OutDataTypeStr=double  OutputDataTypeScalingMode=double  OutDataType=fixdt(0,8)  OutScaling=2^-10
  AC_Res_Profile : simulink/Sources/Repeating Sequence Interpolated  OutValues=[10000 10000 30000 40000 30000 50000 45000 10000]  TimeValues=[0 7 9 11 14 19 22 24]  LookUpMeth=Interpolation-Use End Values  tsamp=0.01  OutMin=[]  OutMax=[]  OutDataTypeStr=double  OutputDataTypeScalingMode=double  OutDataType=fixdt(0,8)  OutScaling=2^-10
  AC_Total : Sum
  Log_Pac : ToWorkspace  VariableName=P_ac_load  SaveFormat=Timeseries  SampleTime=-1
  Log_Pgrid : ToWorkspace  VariableName=P_grid  SaveFormat=Timeseries  SampleTime=-1
  P_grid_ref : Constant  Value=0
  VSC_Idiv : Product  Inputs=*/
  VSC_Isat : Saturate  UpperLimit=200  LowerLimit=-200
  VSC_Ptotal : Sum
  VSC_Vdc_LPF : StateSpace  A=-200  B=200  D=0  InitialCondition=750
  VSC_Vdc_clamp : MinMax  Function=max  Inputs=2
  VSC_Vdc_min : Constant  Value=400
  Out1 : Outport
  Out2 : Outport  Port=2
  wires:
  VSC_Vdc_clamp/1 -> VSC_Idiv/2
  VSC_Vdc_min/1 -> VSC_Vdc_clamp/2
  P_grid_ref/1 -> VSC_Ptotal/2, Log_Pgrid/1
  VSC_Ptotal/1 -> VSC_Idiv/1
  AC_Total/1 -> Out2/1, Log_Pac/1, VSC_Ptotal/1
  VSC_Idiv/1 -> VSC_Isat/1
  AC_Res_Profile/1 -> AC_Total/1
  VSC_Isat/1 -> Out1/1
  AC_Com_Profile/1 -> AC_Total/2
  [Vdc_bus] -> VSC_Vdc_LPF/1
  VSC_Vdc_LPF/1 -> VSC_Vdc_clamp/1

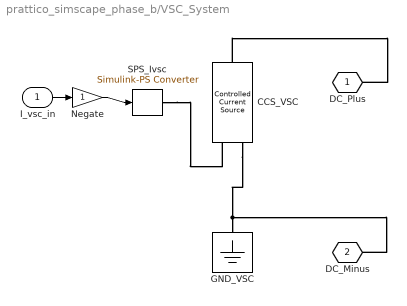
== system prattico_simscape_phase_b/VSC_System ==
  I_vsc_in : Inport
  CCS_VSC : fl_lib/Electrical/Electrical Sources/Controlled Current Source
  GND_VSC : fl_lib/Electrical/Electrical Elements/Electrical Reference
  Negate : Gain
  SPS_Ivsc : nesl_utility/Simulink-PS Converter  PhysicalDomain=network_engine_domain  SubClassName=ps_input  LeftPortType=input  RightPortType=output  PseudoPeriodic=off  Frequencies=[]  NoiseDistribution=none  NoiseParameters=[]  Unit=1  AffineConversion=off  FilteringAndDerivatives=provide  SimscapeFilterOrder=1  InputFilterTimeConstant=0.001  UdotUserProvided=0
  DC_Plus : PMIOPort  Side=Right
  DC_Minus : PMIOPort  Port=2  Side=Right
  wires:
  I_vsc_in/1 -> Negate/1
  Negate/1 -> SPS_Ivsc/1
  connections:
  SPS_Ivsc/RConn1 -- CCS_VSC/RConn1
  CCS_VSC/LConn1 -- DC_Plus/RConn1
  GND_VSC/LConn1 -- CCS_VSC/RConn2 -- DC_Minus/RConn1

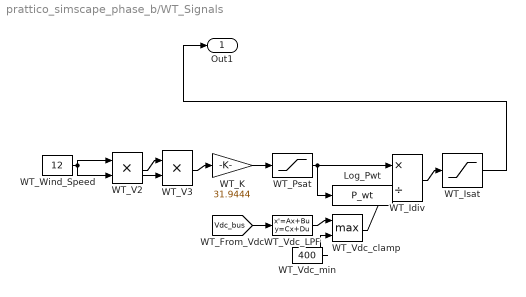
== system prattico_simscape_phase_b/WT_Signals ==
  Log_Pwt : ToWorkspace  VariableName=P_wt  SaveFormat=Timeseries  SampleTime=-1
  WT_Idiv : Product  Inputs=*/
  WT_Isat : Saturate  UpperLimit=150  LowerLimit=0
  WT_K : Gain  Gain=31.9444
  WT_Psat : Saturate  UpperLimit=55200  LowerLimit=0
  WT_V2 : Product  Inputs=**
  WT_V3 : Product  Inputs=**
  WT_Vdc_LPF : StateSpace  A=-200  B=200  D=0  InitialCondition=750
  WT_Vdc_clamp : MinMax  Function=max  Inputs=2
  WT_Vdc_min : Constant  Value=400
  WT_Wind_Speed : Constant  Value=12
  Out1 : Outport
  wires:
  WT_Psat/1 -> Log_Pwt/1, WT_Idiv/1
  WT_V3/1 -> WT_K/1
  WT_Wind_Speed/1 -> WT_V2/1, WT_V2/2, WT_V3/2
  [Vdc_bus] -> WT_Vdc_LPF/1
  WT_V2/1 -> WT_V3/1
  WT_K/1 -> WT_Psat/1
  WT_Vdc_clamp/1 -> WT_Idiv/2
  WT_Idiv/1 -> WT_Isat/1
  WT_Vdc_min/1 -> WT_Vdc_clamp/2
  WT_Vdc_LPF/1 -> WT_Vdc_clamp/1
  WT_Isat/1 -> Out1/1

== system prattico_simscape_phase_b/WT_System ==
  I_wt_in : Inport
  CCS_WT : fl_lib/Electrical/Electrical Sources/Controlled Current Source
  GND_WT : fl_lib/Electrical/Electrical Elements/Electrical Reference
  SPS_Iwt : nesl_utility/Simulink-PS Converter  PhysicalDomain=network_engine_domain  SubClassName=ps_input  LeftPortType=input  RightPortType=output  PseudoPeriodic=off  Frequencies=[]  NoiseDistribution=none  NoiseParameters=[]  Unit=1  AffineConversion=off  FilteringAndDerivatives=provide  SimscapeFilterOrder=1  InputFilterTimeConstant=0.001  UdotUserProvided=0
  DC_Plus : PMIOPort  Side=Right
  DC_Minus : PMIOPort  Port=2  Side=Right
  wires:
  I_wt_in/1 -> SPS_Iwt/1
  connections:
  SPS_Iwt/RConn1 -- CCS_WT/RConn1
  CCS_WT/LConn1 -- DC_Plus/RConn1
  GND_WT/LConn1 -- CCS_WT/RConn2 -- DC_Minus/RConn1
